simulink model "waterlevelsystem"  (R2024b)
settings: Solver=VariableStepAuto  StartTime=0.0  StopTime=100  RelTol=1e-3
settings Model: Creator=Yasara  LastModifiedBy=Yasara

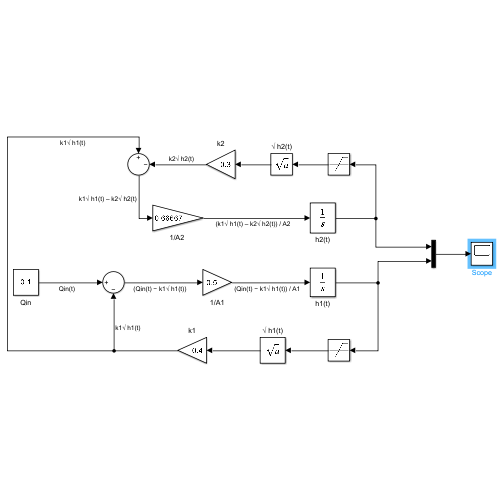
[thumbnail: Simulink's stored preview of the top-level diagram]
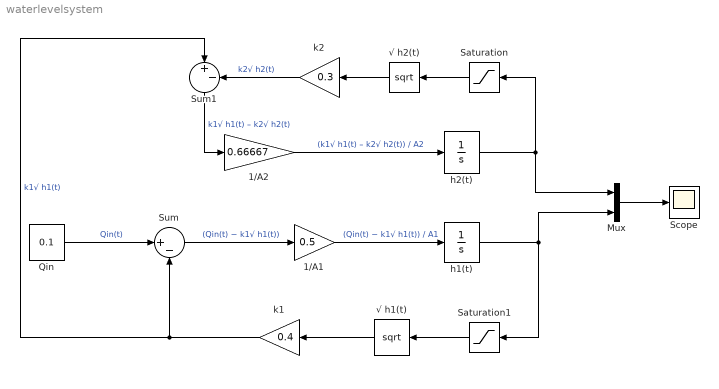
== system waterlevelsystem ==
  1/A1 : Gain  Gain=0.5
  "1/A2 " : Gain  Gain=0.66667
  Mux : Mux  Inputs=2
  Qin : Constant  Value=0.1
  Saturation : Saturate  UpperLimit=inf  LowerLimit=0
  Saturation1 : Saturate  UpperLimit=inf  LowerLimit=0
  Scope : Scope
  Sum : Sum  Inputs=|+-
  Sum1 : Sum  Inputs=|+-
  h1(t) : Integrator
  h2(t) : Integrator
  k1 : Gain  Gain=0.4
  k2 : Gain  Gain=0.3
  √ h1(t) : Sqrt
  √ h2(t) : Sqrt
  wires:
  h1(t)/1 -> Saturation1/1, Mux/2
  Qin/1 -> Sum/1  "Qin(t)"
  h2(t)/1 -> Saturation/1, Mux/1
  √ h2(t)/1 -> k2/1
  k2/1 -> Sum1/2  "k2√ h2(t)"
  Mux/1 -> Scope/1
  k1/1 -> Sum/2, Sum1/1  "k1√ h1(t)"
  √ h1(t)/1 -> k1/1
  1/A1/1 -> h1(t)/1  "(Qin(t) − k1√ h1(t)) / A1"
  Sum/1 -> 1/A1/1  "(Qin(t) − k1√ h1(t))"
  Sum1/1 -> "1/A2 "/1  "k1√ h1(t) – k2√ h2(t)"
  "1/A2 "/1 -> h2(t)/1  "(k1√ h1(t) – k2√ h2(t)) / A2"
  Saturation/1 -> √ h2(t)/1
  Saturation1/1 -> √ h1(t)/1
